simulink model "heli_q8"  (R2025b)
settings: Solver=ode1  StartTime=0.0  StopTime=inf  FixedStep=0.002  RelTol=1e-3  EnableMultiTasking=on
PostLoadFcn:
  | qc_set_target_type(getConfigSet(bdroot, 'QUARC Default Target Configuration'));
undefined symbols (not defined in the file): A_est, B_est, C_est, e_0, F, HIL, Joystick_gain_x, Joystick_gain_y, K, L_obs, P, qc_get_step_size, sw_ecdot, sw_est, sw_pc, t1, t2, t3, t4, Vs_0, x0_obs
libraries: quarc_library x9
settings Model: SimulationMode=external  ExtModeBatchMode=on  ExtModeTrigDuration=30000  Creator=Rchan  LastModifiedBy=alper
settings SolverCC: AlgebraicLoopSolver=TrustRegion  PositivePriorityOrder=on
settings DataIOCC: LimitDataPoints=on  SaveFormat=Array  SignalLoggingSaveFormat=ModelDataLogs  ReturnWorkspaceOutputs=off
settings OptimizationCC: ExpressionDepthLimit=2147483647.0  InitFltsAndDblsToZero=on  LifeSpan=inf
settings DebuggingCC: SaveWithParameterizedLinksMsg=none  UnderspecifiedInitializationDetection=Classic  MergeDetectMultiDrivingBlocksExec=none  SolverPrmCheckMsg=warning  MultiTaskDSMMsg=warning  MultiTaskCondExecSysMsg=none  FcnCallInpInsideContextMsg=warning  UnconnectedInputMsg=warning  UnconnectedOutputMsg=warning  UnconnectedLineMsg=warning  AllowSymbolicDim=off  StateNameClashWarn=warning  SFUnexpectedBacktrackingDiag=warning  SFNoUnconditionalDefaultTransitionDiag=warning  SFExecutionAtInitializationDiag=none  ArithmeticOperatorsInVariantConditions=warning
settings HardwareCC: ProdBitPerPointer=32.0  ProdBitPerSizeT=32.0  ProdBitPerPtrDiffT=32.0  ProdLargestAtomicFloat=None  ProdIntDivRoundTo=Undefined  ProdEndianess=Unspecified  ProdWordSize=32.0  ProdHWDeviceType=32-bit Generic
settings ModelReferenceCC: EnableRefExpFcnMdlSchedulingChecks=on  PropagateSignalLabelsOutOfModel=off
settings SFSimCC: SimUseLocalCustomCode=off  CustomCodeUndefinedFunction=UseInterfaceOnly
settings RTWCC: SystemTargetFile=quarc_win64.tlc  TemplateMakefile=quarc_default_tmf  RTWUseLocalCustomCode=off  GPUComputeCapability=3.5  DLArmComputeVersion=19.05  Description=QUARC Win64 Target
settings CodeAppCC: StateflowObjectComments=on
settings STFCustomTargetCC: SystemTargetFile=quarc_win64.tlc  TargetPreCompLibLocation=C:\PROGRA~3\QUARC\lib\2020b\win64\release  CPPClassGenCompliant=on  StopOnOverrun=off  Debug=off
settings GRTTargetCC: ExtMode=on  ExtModeMexFile=quarc_comm  TargetPreCompLibLocation=C:\PROGRA~3\QUARC\lib\2020b\win64\release  TargetLangStandard=C89/C90 (ANSI)  ParMdlRefBuildCompliant=off  CompOptLevelCompliant=off  CombineOutputUpdateFcns=off  MatFileLogging=off  GRTInterface=on  UseToolchainInfoCompliant=off
settings ConfigComp: CovMetricSettings=dw  CovSaveCumulativeToWorkspaceVar=on  CovSaveSingleToWorkspaceVar=on  CovExternalEMLEnable=off  CovSFcnEnable=off

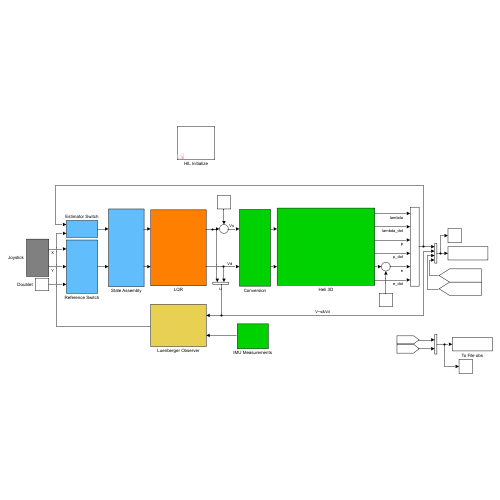
[thumbnail: Simulink's stored preview of the top-level diagram]
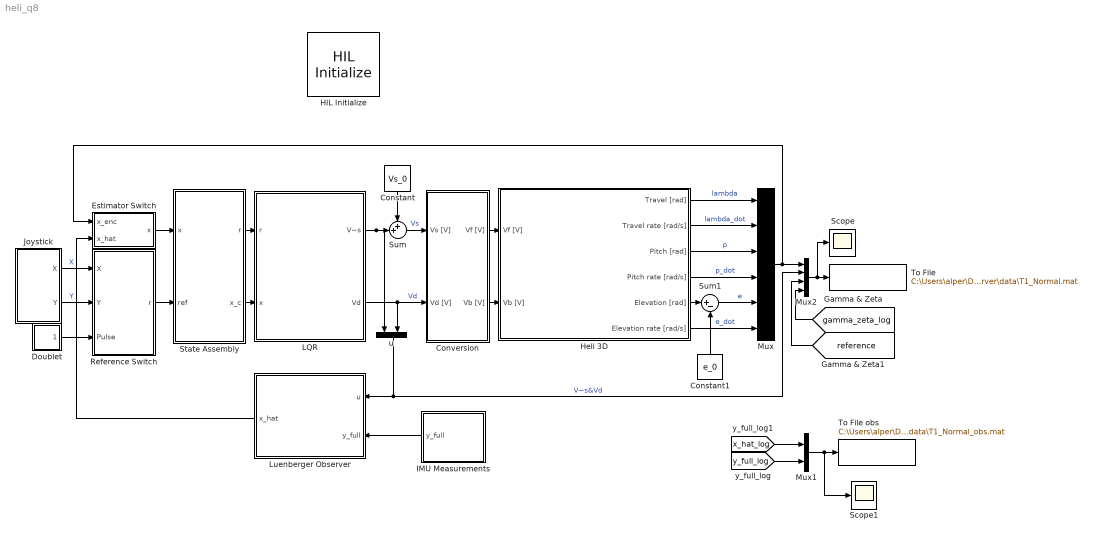
== system heli_q8 ==
  Constant : Constant  Value=Vs_0
  Constant1 : Constant  Value=e_0
  Conversion : Subsystem
  Doublet : Subsystem
  Estimator Switch : Subsystem
  HIL Initialize : quarc_library/Data Acquisition/Generic/Configuration/HIL Initialize  Priority=-99  object_name=HIL-1  board_type=q8_usb  board_number=0  board_options=update_rate=normal;decimation=1  exclusive=off  active=off  hardware_clocks=[0:2]  clock_modes=[]  initial_clock_frequencies=[]  set_clock_params_at_start=off  set_clock_params_at_switch_in=off  set_clock_frequencies_at_start=off  set_clock_frequencies_at_switch_in=off  analog_input_channels=[0:7]  analog_input_configurations=[]  analog_input_maximums=10  analog_input_minimums=-10  set_analog_input_params_at_start=on  set_analog_input_params_at_switch_in=off  analog_output_channels=[0:7]  analog_output_maximums=10  analog_output_minimums=-10  initial_analog_outputs=[0]  final_analog_outputs=[0]  watchdog_analog_outputs=0  set_analog_output_params_at_start=on  set_analog_output_params_at_switch_in=off  set_analog_outputs_at_start=on  set_analog_outputs_at_switch_in=off  set_analog_outputs_at_terminate=on  set_analog_outputs_at_switch_out=off  set_analog_outputs_on_watchdog=off  digital_input_channels=[]  digital_output_channels=[]  digital_output_configuration=[]  initial_digital_outputs=[1]  final_digital_outputs=[1]  watchdog_digital_outputs=[1]  set_digital_output_params_at_start=off  set_digital_output_params_at_switch_in=off  set_digital_outputs_at_start=on  set_digital_outputs_at_switch_in=off  set_digital_outputs_at_terminate=on  set_digital_outputs_at_switch_out=off  set_digital_outputs_on_watchdog=off  encoder_channels=[0:7]  quadrature=[4]  encoder_filter_frequency=[]  initial_encoder_counts=[0]  set_encoder_params_at_start=on  set_encoder_params_at_switch_in=off  set_encoder_counts_at_start=on  set_encoder_counts_at_switch_in=off  pwm_channels=[0:7]  pwm_modes=0  pwm_frequency=99.532799999999995e6/4095  pwm_configuration=[0]  pwm_alignment=[0]  pwm_polarity=[1]  pwm_leading_deadband=[0]  pwm_trailing_deadband=[0]  initial_pwm_outputs=[0]  final_pwm_outputs=[0]  watchdog_pwm_outputs=[0]  set_pwm_params_at_start=on  set_pwm_params_at_switch_in=off  set_pwm_outputs_at_start=on  set_pwm_outputs_at_switch_in=off  set_pwm_outputs_at_terminate=on  set_pwm_outputs_at_switch_out=off  set_pwm_outputs_on_watchdog=off  other_output_channels=[]  initial_other_outputs=[]  final_other_outputs=[]  watchdog_other_outputs=[]  set_other_outputs_at_start=off  set_other_outputs_at_switch_in=off  set_other_outputs_at_terminate=off  set_other_outputs_at_switch_out=off  set_other_outputs_on_watchdog=off
  Heli 3D : Subsystem
  IMU Measurements : Subsystem
      settings: PortSchema="{\"entries\":[{\"content\":{\"sides\":[{\"content\":{\"connectorIds\":[\"Out1\"]},\"type\":\"ConnectorPlacement.EquallySpacedRectSide\",\"uuid\":\"f2c6d1a5-b23e-49f7-b327-3ce99357b705\"},{\"content\":{\"side\":\"RIGHT\"},\"type\":\"ConnectorPlacement.EquallySpacedRectSide\",\"uuid\":\"fa4197e5-e45b-49ac-a739-44a65bd19529\"},{\"content\":{\"side\":\"TOP\"},\"type\":\"ConnectorPlacement.EquallySpacedRectSide\",\"uuid\":\"393299b5-98b8-4f5f-8969-df60afad8ba6\"}]},\"type\":\"ConnectorPlacement.EquallySpacedConnector\",\"uuid\":\"350d1e40-a133-4cdf-a2d9-3eea3343136e\"}],\"packageUris\":[\"http://schema.mathworks.com/mf0/Connector/R2020b\"],\"version\":\"1.0\"}"
  Joystick : Subsystem
  LQR : Subsystem
  Luenberger Observer : Subsystem
  Mux : Mux  Inputs=6
  Mux1 : Mux  Inputs=2
  Mux2 : Mux
  Reference Switch : Subsystem
  Scope : Scope
      settings: ActiveDisplayYMinimum=-3.57999  ActiveDisplayYMaximum=28.38185
  Scope1 : Scope
      settings: ActiveDisplayYMinimum=-3.57999  ActiveDisplayYMaximum=28.38185
  State Assembly : Subsystem
  Sum : Sum  Inputs=++|
  Sum1 : Sum  Inputs=|+-
  To File : ToFile  Filename=C:\Users\alper\Documents\H26\Linsys\Helicopter-lab\Task 3.3 - Observer\data\T1_Normal.mat  MatrixName=heli_log
  To File obs : ToFile  Filename=C:\Users\alper\Documents\H26\Linsys\Helicopter-lab\Task 3.3 - Observer\data\T1_Normal_obs.mat  MatrixName=obs_log
  u : Mux  Inputs=2
  wires:
  Conversion/2(Vb [V]) -> Heli 3D/2(Vb [V])
  Conversion/1(Vf [V]) -> Heli 3D/1(Vf [V])
  Heli 3D/1(Travel [rad]) -> Mux/1  "lambda"
  Heli 3D/2(Travel rate [rad/s]) -> Mux/2  "lambda_dot"
  Heli 3D/4(Pitch rate [rad/s]) -> Mux/4  "p_dot"
  Heli 3D/6(Elevation rate [rad/s]) -> Mux/6  "e_dot"
  Sum/1 -> Conversion/1(Vs [V])  "Vs"
  Heli 3D/5(Elevation [rad]) -> Sum1/1
  Sum1/1 -> Mux/5  "e"
  Constant1/1 -> Sum1/2
  Heli 3D/3(Pitch [rad]) -> Mux/3  "p"
  Constant/1 -> Sum/1
  LQR/1(V~s) -> u/1, Sum/2
  State Assembly/1(r) -> LQR/1(r)
  LQR/2(Vd) -> u/2, Conversion/2(Vd [V])  "Vd"
  Mux/1 -> Estimator Switch/1(x_enc), Mux2/1
  Joystick/2(Y) -> Reference Switch/2(Y)  "Y"
  Mux2/1 -> Scope/1, To File/1
  u/1 -> Mux2/2, Luenberger Observer/1(u)  "V~s&Vd"
  Joystick/1(X) -> Reference Switch/1(X)  "X"
  [reference] -> Mux2/3
  [gamma_zeta_log] -> Mux2/4
  IMU Measurements/1(y_full) -> Luenberger Observer/2(y_full)
  Doublet/1(Out1) -> Reference Switch/3(Pulse)
  Luenberger Observer/1(x_hat) -> Estimator Switch/2(x_hat)
  Reference Switch/1(r) -> State Assembly/2(ref)
  Estimator Switch/1(x) -> State Assembly/1(x)
  State Assembly/2(x_c) -> LQR/2(x)
  Mux1/1 -> Scope1/1, To File obs/1
  [y_full_log] -> Mux1/2
  [x_hat_log] -> Mux1/1

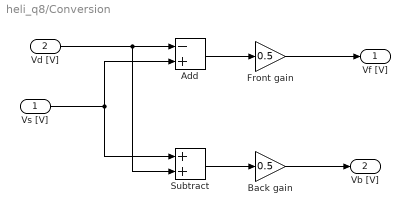
== system heli_q8/Conversion ==
  Vs [V] : Inport
  Vd [V] : Inport  Port=2
  Add : Sum  Inputs=-+
  Back gain : Gain  Gain=0.5
  Front gain : Gain  Gain=0.5
  Subtract : Sum
  Vf [V] : Outport
  Vb [V] : Outport  Port=2
  wires:
  Vd [V]/1 -> Subtract/2, Add/1
  Vs [V]/1 -> Subtract/1, Add/2
  Subtract/1 -> Back gain/1
  Back gain/1 -> Vb [V]/1
  Add/1 -> Front gain/1
  Front gain/1 -> Vf [V]/1

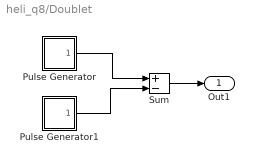
== system heli_q8/Doublet ==
  Pulse Generator : Subsystem
  Pulse Generator1 : Subsystem
  Sum : Sum  Inputs=+-
  Out1 : Outport
  wires:
  Sum/1 -> Out1/1
  Pulse Generator/1(Pulse) -> Sum/1
  Pulse Generator1/1(Pulse) -> Sum/2

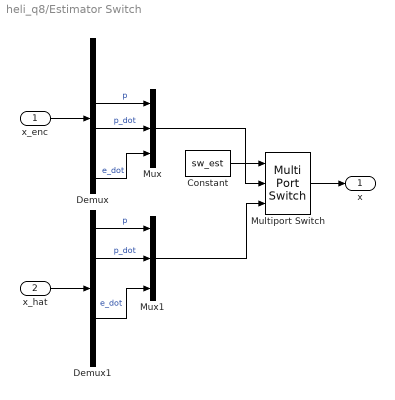
== system heli_q8/Estimator Switch ==
  x_enc : Inport
  x_hat : Inport  Port=2
  Constant : Constant  Value=sw_est
  Demux : Demux  Outputs=6
  Demux1 : Demux  Outputs=5
  Multiport Switch : MultiPortSwitch  DataPortOrder=Zero-based contiguous  Inputs=2  zeroidx=on  SaturateOnIntegerOverflow=off  InputSameDT=off
  Mux : Mux  Inputs=3
  Mux1 : Mux  Inputs=3
  x : Outport
  wires:
  x_enc/1 -> Demux/1
  Demux/3 -> Mux/1  "p"
  Demux/4 -> Mux/2  "p_dot"
  Demux/6 -> Mux/3  "e_dot"
  Mux/1 -> Multiport Switch/2
  x_hat/1 -> Demux1/1
  Multiport Switch/1 -> x/1
  Constant/1 -> Multiport Switch/1
  Demux1/1 -> Mux1/1  "p"
  Demux1/2 -> Mux1/2  "p_dot"
  Demux1/4 -> Mux1/3  "e_dot"
  Mux1/1 -> Multiport Switch/3

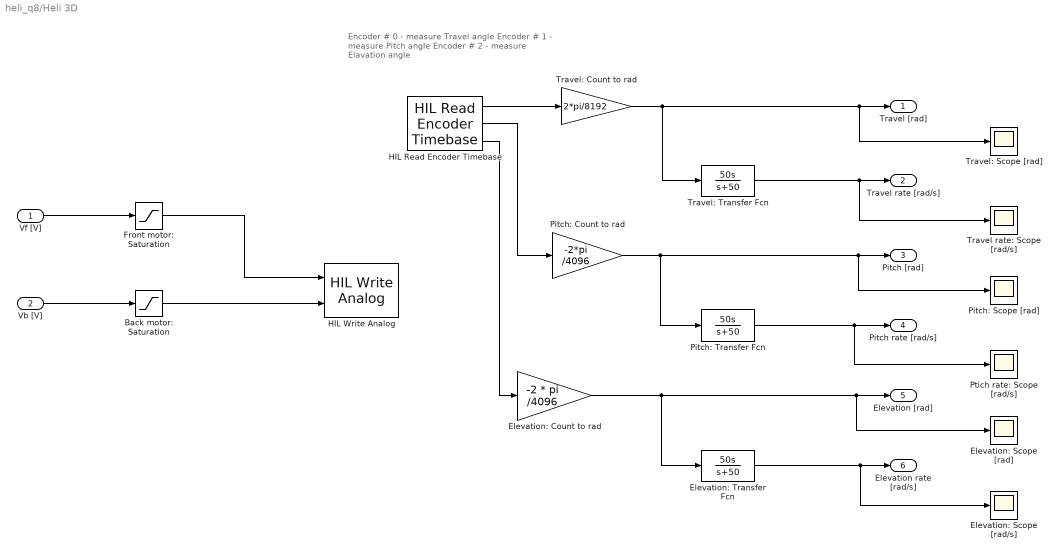
== system heli_q8/Heli 3D ==
  note: Encoder # 0 - measure Travel angle
      | Encoder # 1 - measure Pitch angle
      | Encoder # 2 - measure Elavation angle
  Vf [V] : Inport
  Vb [V] : Inport  Port=2
  Back motor: Saturation : Saturate  UpperLimit=5  LowerLimit=-5
  Elevation: Count to rad : Gain  Gain=-2 * pi /4096
  Elevation: Scope [rad/s] : Scope
      settings: ActiveDisplayYMinimum=-15  ActiveDisplayYMaximum=15  DataLoggingVariableName=ScopeData13
  Elevation: Scope [rad] : Scope
      settings: ActiveDisplayYMinimum=0.52213  ActiveDisplayYMaximum=0.53172  DataLoggingVariableName=ScopeData12
  Elevation: Transfer Fcn : TransferFcn  Numerator=[50 0]  Denominator=[1 50]
  Front motor: Saturation : Saturate  UpperLimit=5  LowerLimit=-5
  HIL Read Encoder Timebase : quarc_library/Data Acquisition/Generic/Timebases/HIL Read Encoder Timebase  object_name=HIL-1  clock=0  channels=[0:2]  active=on  vector_output=off  data_type_mode=Inherit via back propagation  data_type=double  overflow_mode=Error on overflow  samples_in_buffer=max(ceil(1/qc_get_step_size), 1)
  HIL Write Analog : quarc_library/Data Acquisition/Generic/Immediate I//O/HIL Write Analog  object_name=HIL-1  channels=[0:1]  sample_time=-1  active=off  vector_input=off
  Pitch: Count to rad : Gain  Gain=-2*pi /4096
  Pitch: Scope [rad] : Scope
      settings: ActiveDisplayYMinimum=-15  ActiveDisplayYMaximum=15  DataLoggingVariableName=ScopeData10
  Pitch: Transfer Fcn : TransferFcn  Numerator=[50 0]  Denominator=[1 50]
  Ptich rate: Scope [rad/s] : Scope
      settings: ActiveDisplayYMinimum=-15  ActiveDisplayYMaximum=15  DataLoggingVariableName=ScopeData11
  Travel rate: Scope [rad/s] : Scope
      settings: ActiveDisplayYMinimum=-15  ActiveDisplayYMaximum=15  DataLoggingVariableName=ScopeData9
  Travel: Count to rad : Gain  Gain=2*pi/8192
  Travel: Scope [rad] : Scope
      settings: ActiveDisplayYMinimum=-15  ActiveDisplayYMaximum=15  DataLoggingVariableName=ScopeData8
  Travel: Transfer Fcn : TransferFcn  Numerator=[50 0]  Denominator=[1 50]
  Travel [rad] : Outport
  Travel rate [rad/s] : Outport  Port=2
  Pitch [rad] : Outport  Port=3
  Pitch rate [rad/s] : Outport  Port=4
  Elevation [rad] : Outport  Port=5
  Elevation rate [rad/s] : Outport  Port=6
  wires:
  HIL Read Encoder Timebase/1 -> Travel: Count to rad/1
  HIL Read Encoder Timebase/2 -> Pitch: Count to rad/1
  HIL Read Encoder Timebase/3 -> Elevation: Count to rad/1
  Travel: Count to rad/1 -> Travel: Scope [rad]/1, Travel [rad]/1, Travel: Transfer Fcn/1
  Travel: Transfer Fcn/1 -> Travel rate: Scope [rad/s]/1, Travel rate [rad/s]/1
  Pitch: Count to rad/1 -> Pitch: Transfer Fcn/1, Pitch: Scope [rad]/1, Pitch [rad]/1
  Pitch: Transfer Fcn/1 -> Ptich rate: Scope [rad/s]/1, Pitch rate [rad/s]/1
  Elevation: Count to rad/1 -> Elevation: Transfer Fcn/1, Elevation: Scope [rad]/1, Elevation [rad]/1
  Elevation: Transfer Fcn/1 -> Elevation: Scope [rad/s]/1, Elevation rate [rad/s]/1
  Vf [V]/1 -> Front motor: Saturation/1
  Vb [V]/1 -> Back motor: Saturation/1
  Front motor: Saturation/1 -> HIL Write Analog/1
  Back motor: Saturation/1 -> HIL Write Analog/2

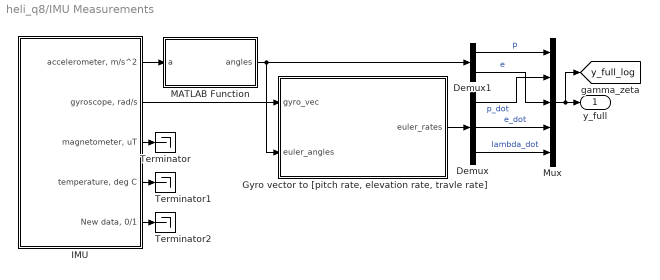
== system heli_q8/IMU Measurements ==
  Demux : Demux  Outputs=3
  Demux1 : Demux  Outputs=2
  "Gyro vector to [pitch rate, elevation rate, travle rate]" : MATLAB Function  TreatAsAtomicUnit=on
  IMU : Subsystem
  MATLAB Function : MATLAB Function  TreatAsAtomicUnit=on
  Mux : Mux  Inputs=5
  Terminator : Terminator
  Terminator1 : Terminator
  Terminator2 : Terminator
  y_full : Outport
  tag scope: y_full_log=global
  wires:
  IMU/2("gyroscope, rad/s") -> "Gyro vector to [pitch rate, elevation rate, travle rate]"/1(gyro_vec)
  IMU/1("accelerometer, m/s^2") -> MATLAB Function/1(a)
  MATLAB Function/1(angles) -> "Gyro vector to [pitch rate, elevation rate, travle rate]"/2(euler_angles), Demux1/1
  "Gyro vector to [pitch rate, elevation rate, travle rate]"/1(euler_rates) -> Demux/1
  Mux/1 -> [y_full_log], y_full/1
  Demux1/1 -> Mux/1  "p"
  Demux/1 -> Mux/2  "p_dot"
  Demux1/2 -> Mux/3  "e"
  Demux/2 -> Mux/4  "e_dot"
  Demux/3 -> Mux/5  "lambda_dot"
  IMU/3("magnetometer, uT") -> Terminator/1
  IMU/4("temperature, deg C") -> Terminator1/1
  IMU/5("New data, 0/1") -> Terminator2/1

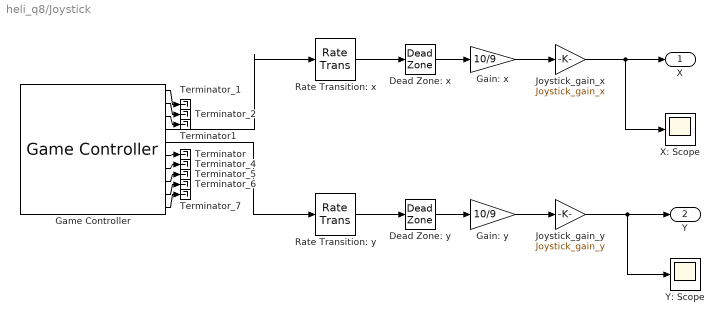
== system heli_q8/Joystick ==
  Dead Zone: x : DeadZone  LowerValue=-0.1  UpperValue=0.1
  Dead Zone: y : DeadZone  LowerValue=-0.1  UpperValue=0.1
  Gain: x : Gain  Gain=10/9
  Gain: y : Gain  Gain=10/9
  Game Controller : quarc_library/Devices/Peripherals/Target/Game Controller  controller=1  buffer_size=12  deadzone=[]  saturation=[]  sample_time=max(qc_get_step_size, 0.01)  auto_center=off  enabled=on
      settings: SourceProductName=QUARC Targets
  Joystick_gain_x : Gain  Gain=Joystick_gain_x
  Joystick_gain_y : Gain  Gain=Joystick_gain_y
  Rate Transition: x : RateTransition
  Rate Transition: y : RateTransition
  Terminator : Terminator
  Terminator1 : Terminator
  Terminator_{1..2,4..7} (6 alike) : Terminator
  X: Scope : Scope
      settings: ActiveDisplayYMinimum=-1  ActiveDisplayYMaximum=1  DataLoggingVariableName=ScopeData7
  Y: Scope : Scope
      settings: DataLoggingVariableName=ScopeData5
  X : Outport
  Y : Outport  Port=2
  wires:
  Rate Transition: y/1 -> Dead Zone: y/1
  Rate Transition: x/1 -> Dead Zone: x/1
  Game Controller/5 -> Rate Transition: y/1
  Game Controller/4 -> Rate Transition: x/1
  Game Controller/1 -> Terminator_1/1
  Game Controller/2 -> Terminator_2/1
  Game Controller/7 -> Terminator_4/1
  Game Controller/8 -> Terminator_5/1
  Game Controller/9 -> Terminator_6/1
  Game Controller/10 -> Terminator_7/1
  Game Controller/3 -> Terminator1/1
  Game Controller/6 -> Terminator/1
  Dead Zone: x/1 -> Gain: x/1
  Dead Zone: y/1 -> Gain: y/1
  Gain: x/1 -> Joystick_gain_x/1
  Gain: y/1 -> Joystick_gain_y/1
  Joystick_gain_x/1 -> X/1, X: Scope/1
  Joystick_gain_y/1 -> Y: Scope/1, Y/1

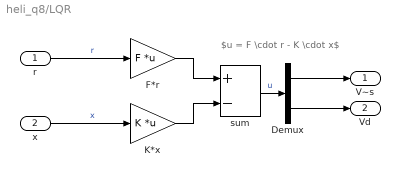
== system heli_q8/LQR ==
  note: $u = F \cdot r - K \cdot x$
  r : Inport
  x : Inport  Port=2
  Demux : Demux  Outputs=2
  F*r : Gain  Gain=F  Multiplication=Matrix(K*u)
  K*x : Gain  Gain=K  Multiplication=Matrix(K*u)
  sum : Sum  Inputs=+-
  V~s : Outport
  Vd : Outport  Port=2
  wires:
  r/1 -> F*r/1  "r"
  F*r/1 -> sum/1
  K*x/1 -> sum/2
  sum/1 -> Demux/1  "u"
  Demux/1 -> V~s/1
  Demux/2 -> Vd/1
  x/1 -> K*x/1  "x"

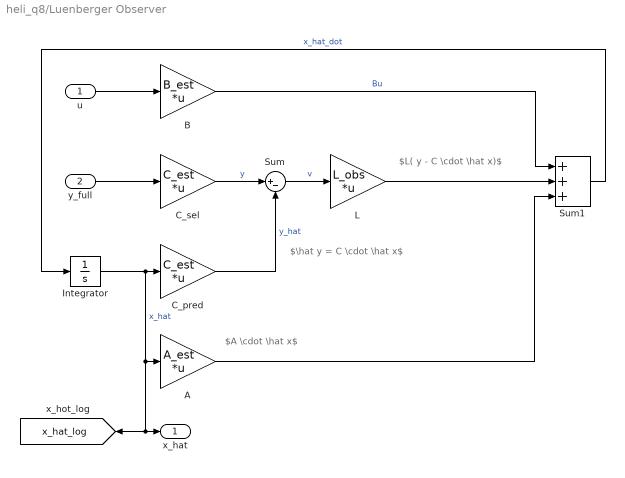
== system heli_q8/Luenberger Observer ==
  note: $\hat y = C \cdot \hat x$
  note: $L( y - C \cdot \hat x)$
  note: $A \cdot \hat x$
  u : Inport
  y_full : Inport  Port=2
  A : Gain  Gain=A_est  Multiplication=Matrix(K*u)
  B : Gain  Gain=B_est  Multiplication=Matrix(K*u)
  C_pred : Gain  Gain=C_est  Multiplication=Matrix(K*u)
  C_sel : Gain  Gain=C_est  Multiplication=Matrix(K*u)
  Integrator : Integrator  InitialCondition=x0_obs
  L : Gain  Gain=L_obs  Multiplication=Matrix(K*u)
  Sum : Sum  Inputs=|+-
  Sum1 : Sum  Inputs=+|+|+
  x_hat : Outport
  tag scope: x_hat_log=global
  wires:
  y_full/1 -> C_sel/1
  C_sel/1 -> Sum/1  "y"
  C_pred/1 -> Sum/2  "y_hat"
  Sum/1 -> L/1  "v"
  Integrator/1 -> x_hat/1, [x_hat_log], A/1, C_pred/1  "x_hat"
  u/1 -> B/1
  B/1 -> Sum1/1  "Bu"
  Sum1/1 -> Integrator/1  "x_hat_dot"
  A/1 -> Sum1/3
  L/1 -> Sum1/2

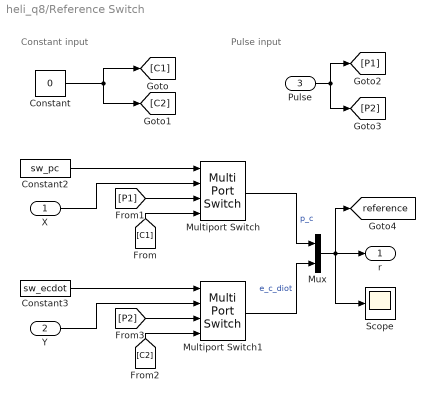
== system heli_q8/Reference Switch ==
  note: Pulse input
  note: Constant input
  X : Inport
  Y : Inport  Port=2
  Pulse : Inport  Port=3
  Constant : Constant  Value=0
  Constant2 : Constant  Value=sw_pc
  Constant3 : Constant  Value=sw_ecdot
  Multiport Switch : MultiPortSwitch  SaturateOnIntegerOverflow=off  InputSameDT=off
  Multiport Switch1 : MultiPortSwitch  SaturateOnIntegerOverflow=off  InputSameDT=off
  Mux : Mux  Inputs=2
  Scope : Scope
      settings: ActiveDisplayYMinimum=-1  ActiveDisplayYMaximum=1
  r : Outport
  tag scope: reference=global
  wires:
  Mux/1 -> Scope/1, r/1, [reference]
  Multiport Switch/1 -> Mux/1  "p_c"
  X/1 -> Multiport Switch/2
  Constant/1 -> [C2], [C1]
  Pulse/1 -> [P2], [P1]
  [C1] -> Multiport Switch/4
  [P1] -> Multiport Switch/3
  [P2] -> Multiport Switch1/3
  Constant3/1 -> Multiport Switch1/1
  Y/1 -> Multiport Switch1/2
  [C2] -> Multiport Switch1/4
  Multiport Switch1/1 -> Mux/2  "e_c_diot"
  Constant2/1 -> Multiport Switch/1

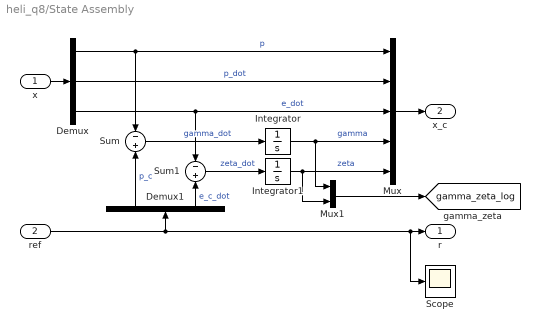
== system heli_q8/State Assembly ==
  x : Inport
  ref : Inport  Port=2
  Demux : Demux  Outputs=3
  Demux1 : Demux  Outputs=2
  Integrator : Integrator
  Integrator1 : Integrator  InitialCondition=e_0
  Mux : Mux  Inputs=5
  Mux1 : Mux  Inputs=2
  Scope : Scope
      settings: ActiveDisplayYMinimum=-1  ActiveDisplayYMaximum=1
  Sum : Sum  Inputs=-|+
  Sum1 : Sum  Inputs=-|+
  r : Outport
  x_c : Outport  Port=2
  tag scope: gamma_zeta_log=global
  wires:
  ref/1 -> Scope/1, r/1, Demux1/1
  Demux1/1 -> Sum/2  "p_c"
  Demux/1 -> Sum/1, Mux/1  "p"
  Sum/1 -> Integrator/1  "gamma_dot"
  Demux1/2 -> Sum1/2  "e_c_dot"
  Demux/3 -> Sum1/1, Mux/3  "e_dot"
  Sum1/1 -> Integrator1/1  "zeta_dot"
  Mux/1 -> x_c/1
  Integrator1/1 -> Mux/5, Mux1/2  "zeta"
  Integrator/1 -> Mux1/1, Mux/4  "gamma"
  Demux/2 -> Mux/2  "p_dot"
  Mux1/1 -> [gamma_zeta_log]
  x/1 -> Demux/1

== system heli_q8/Doublet/Pulse Generator ==
  First : Step  Time=t1  After=P  SampleTime=0
  Second : Step  Time=t2  After=-P  SampleTime=0
  Sum : Sum
  Pulse : Outport
  wires:
  Sum/1 -> Pulse/1
  Second/1 -> Sum/2
  First/1 -> Sum/1

== system heli_q8/Doublet/Pulse Generator1 ==
  First : Step  Time=t3  After=P  SampleTime=0
  Second : Step  Time=t4  After=-P  SampleTime=0
  Sum : Sum
  Pulse : Outport
  wires:
  Sum/1 -> Pulse/1
  Second/1 -> Sum/2
  First/1 -> Sum/1

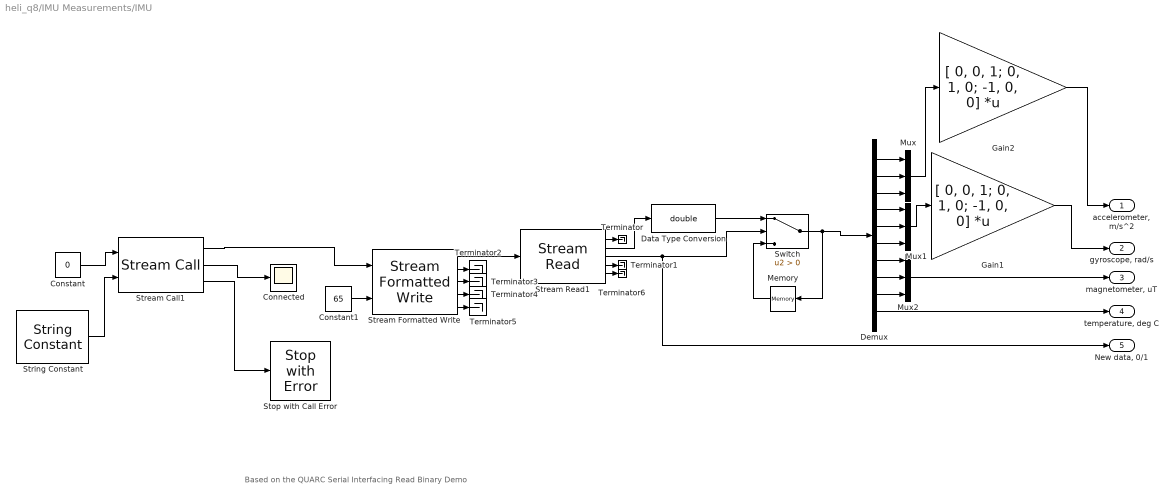
== system heli_q8/IMU Measurements/IMU ==
  note: Based on the QUARC Serial Interfacing Read Binary Demo
  Connected : Scope
      settings: DataLoggingVariableName=ScopeData6
  Constant : Constant  Value=0
  Constant1 : Constant  Value=65
  Data Type Conversion : DataTypeConversion  OutDataTypeStr=double  SaturateOnIntegerOverflow=off  RndMeth=Floor
  Demux : Demux  Outputs=10
  Gain1 : Gain  Gain=[ 0, 0, 1; 0, 1, 0; -1, 0, 0]  Multiplication=Matrix(K*u) (u vector)
  Gain2 : Gain  Gain=[ 0, 0, 1; 0, 1, 0; -1, 0, 0]  Multiplication=Matrix(K*u) (u vector)
  Memory : Memory  InitialCondition=[0 0 0 0 0 0 0 0 0 0]
  Mux : Mux  Inputs=3
  Mux1 : Mux  Inputs=3
  Mux2 : Mux  Inputs=3
  Stop with Call Error : quarc_library/Sinks/Error Handling/Stop with Error  message_type=Interpret input as error code  message=Error occurred
      settings: SourceProductName=QUARC Targets
  Stream Call1 : quarc_library/Communications/Intermediate/Stream Call  uri_source=External input port  uri=serial://IMU:9?baud=115200,word=8,parity=none,stop=1,flow='none'  apply_uri_to_all_configs=on  send_buffer_size=8000  receive_buffer_size=8000  byte_order=little endian (Intel - LSB first)  sample_time=qc_get_step_size  non_blocking=on  active=off
      settings: SourceProductName=QUARC Targets
  Stream Formatted Write : quarc_library/Communications/Intermediate/Stream Formatted Write  format_string=%c\n  max_code_units=80  optimization=Minimizing latency
      settings: SourceProductName=QUARC Targets
  Stream Read1 : quarc_library/Communications/Intermediate/Stream Read  data_type=single  type_expr=BusObject  num_elements=10  receive_dims=off
      settings: SourceProductName=QUARC Targets
  String Constant : quarc_library/Strings/String Constant  string_value=qc_perform_substitutions('serial://IMU:%{PORT}?baud=115200,word=8,parity=none,stop=1')  evaluate_string=on  string_type=URI  max_length=255  sample_time=inf  variable_size=off
      settings: AttributesFormatString="\"serial://IMU:%{PORT}?baud=115200,word=8,parity=none,stop=1\""  SourceProductName=QUARC Targets
  Switch : Switch  Criteria=u2 > Threshold  SaturateOnIntegerOverflow=off  InputSameDT=off
  Terminator{,1..6} (7 alike) : Terminator
  "accelerometer, m/s^2" : Outport
  "gyroscope, rad/s" : Outport  Port=2
  "magnetometer, uT" : Outport  Port=3
  "temperature, deg C" : Outport  Port=4
  "New data, 0/1" : Outport  Port=5
  wires:
  Switch/1 -> Memory/1, Demux/1
  Data Type Conversion/1 -> Switch/1
  Stream Read1/3 -> "New data, 0/1"/1, Switch/2
  Stream Formatted Write/1 -> Stream Read1/1
  Constant1/1 -> Stream Formatted Write/2
  Gain1/1 -> "gyroscope, rad/s"/1
  Gain2/1 -> "accelerometer, m/s^2"/1
  Stream Read1/4 -> Terminator1/1
  Demux/10 -> "temperature, deg C"/1
  Mux1/1 -> Gain1/1
  Stream Read1/2 -> Data Type Conversion/1
  Demux/7 -> Mux2/1
  Demux/8 -> Mux2/2
  Demux/9 -> Mux2/3
  Mux2/1 -> "magnetometer, uT"/1
  Demux/6 -> Mux1/3
  Demux/5 -> Mux1/2
  Demux/4 -> Mux1/1
  Mux/1 -> Gain2/1
  Demux/3 -> Mux/3
  Demux/1 -> Mux/1
  Demux/2 -> Mux/2
  Stream Read1/1 -> Terminator/1
  Stream Call1/1 -> Stream Formatted Write/1
  Constant/1 -> Stream Call1/1
  String Constant/1 -> Stream Call1/2
  Stream Call1/2 -> Connected/1
  Stream Call1/3 -> Stop with Call Error/1
  Memory/1 -> Switch/3
  Stream Formatted Write/2 -> Terminator2/1
  Stream Formatted Write/3 -> Terminator3/1
  Stream Formatted Write/4 -> Terminator4/1
  Stream Formatted Write/5 -> Terminator5/1
  Stream Read1/5 -> Terminator6/1

== matlab function heli_q8/IMU Measurements/Gyro vector to [pitch rate, elevation rate, travle rate] ==
  data: gyro_vec input; euler_rates output; euler_angles input
function euler_rates = gyro_vec_to_euler_rates(gyro_vec,euler_angles)
%#codegen
    phi = euler_angles(1);
    theta = euler_angles(2);


    T = [1, sin(phi)*tan(theta), cos(phi)*tan(theta);
         0, cos(phi),            -sin(phi);
         0, sin(phi)/cos(theta), cos(phi)/cos(theta)]; 
euler_rates = T*gyro_vec;

== matlab function heli_q8/IMU Measurements/MATLAB Function ==
  data: a input; angles output
function angles = acc_to_angles(a)
% a      : [ax; ay; az]
% angles : [pitch; elevation] 

ax = a(1);  ay = a(2);  az = a(3);

if ax == 0 && ay == 0 && az == 0     % startup
    angles = [0; 0];
    return
end

p = atan2(-ay, -az);                 
e = atan2(ax, sqrt(ay^2 + az^2));     
angles = [p; e];
end
